simulink model "Modelo_Sensores_Ancho_banda_limitado"  (R2017a)
settings: Solver=VariableStepAuto  StartTime=0.0  StopTime=25  RelTol=1e-3
values from neighbouring files (symbols this model uses):
  alfa_cu = 3.9e-3    (= 0.0039)    [modelo_global_NL.m]
  ba = Jeq*n*wpos    (= 0.0113117692401)    [modelo_global_NL.m]
  beq = bl/r^2 + bm    (= 1.5638971155e-05)    [Evaluacion_polos_5_2_2.m]    (also in modelo_global_NL.m = 1.5e-05)
  Cts = 0.818    [modelo_global_NL.m]
  den_iabc = [1 2*wn_iabc*xita_iabc wn_iabc^2]    [modelo_global_NL.m]
  den_t = [1 2*wn_t*xita_t wn_t^2]    [modelo_global_NL.m]
  den_temp = [tau 1]    [modelo_global_NL.m]
  Jeq = Jl/r^2 + Jm    (= 6.9338269301e-06)    [Evaluacion_polos_5_2_2.m]    (also in modelo_global_NL.m = 5.65588462007e-06)
  ki = 6.5536e10    (= 65536000000)    [modelo_global_NL.m]
  Ksa = Jeq*n*wpos^2    (= 9.04941539211)    [modelo_global_NL.m]
  Ksia = Jeq*wpos^3    (= 2895.81292547)    [modelo_global_NL.m]
  kt = 12800    [modelo_global_NL.m]
  kw = 5.12e7    (= 51200000)    [modelo_global_NL.m]
  LambdaM = 0.01546    [Evaluacion_polos_5_2_2.m]    (also in modelo_global_NL.m)
  Ld = 0.0066    [Evaluacion_polos_5_2_2.m]    (also in modelo_global_NL.m)
  Lq = 0.0058    [Evaluacion_polos_5_2_2.m]    (also in modelo_global_NL.m)
  num_iabc = [wn_iabc^2]    [modelo_global_NL.m]
  num_t = [wn_t^2]    [modelo_global_NL.m]
  num_temp = [1]    [modelo_global_NL.m]
  Pp = 3    [Evaluacion_polos_5_2_2.m]    (also in modelo_global_NL.m)
  r = 314    [Evaluacion_polos_5_2_2.m]    (also in modelo_global_NL.m)
  R0 = 4    [Evaluacion_polos_5_2_2.m]    (also in modelo_global_NL.m)
  Rd = 33    [Evaluacion_polos_5_2_2.m]    (also in modelo_global_NL.m)
  Rq = 29    [Evaluacion_polos_5_2_2.m]    (also in modelo_global_NL.m)
  Rs = 1.02    [Evaluacion_polos_5_2_2.m]    (also in modelo_global_NL.m)
  Rsref = 1.02    [modelo_global_NL.m]
  Rts_amb = 146.7    [modelo_global_NL.m]
  Tamb = 40    [modelo_global_NL.m]
  Tleq = Tl/r    (= 0.02)    [modelo_global_NL.m]
  Tsref = 40    [modelo_global_NL.m]
undefined symbols (not defined in the file or in its folder): sigbuilder_block
settings Model: Creator=merem  LastModifiedBy=merem

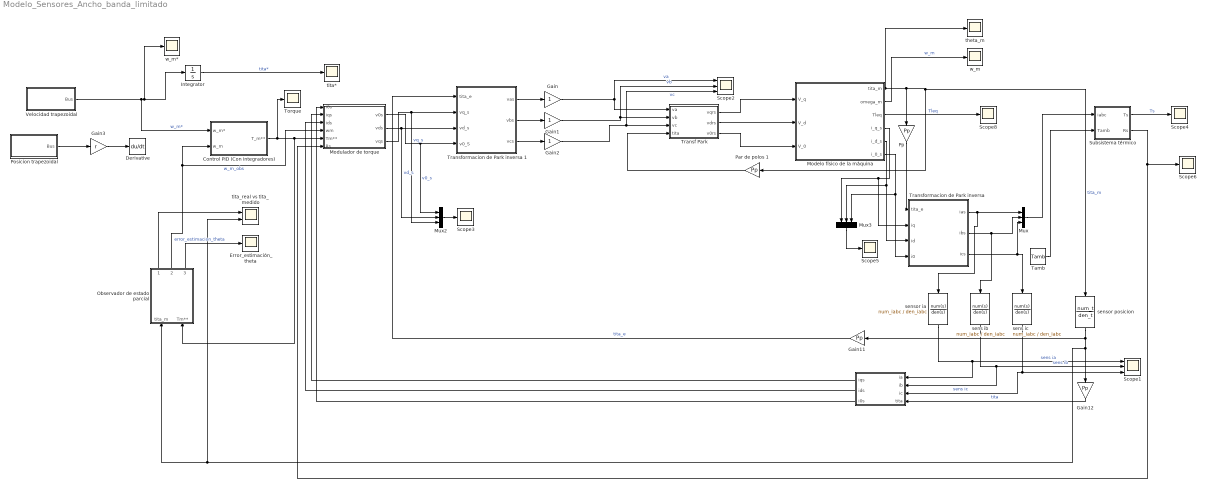
== system Modelo_Sensores_Ancho_banda_limitado ==
  " " : Subsystem
  Control PID (Con integradores) : Subsystem
  Derivative : Derivative
  Error_estimación_theta : Scope
  Gain : Gain
  Gain1 : Gain
  Gain11 : Gain  Gain=Pp
  Gain12 : Gain  Gain=Pp
  Gain2 : Gain
  Gain3 : Gain  Gain=r
  Integrator : Integrator
  Modelo físico de la máquina : Subsystem
  Modulador de torque : Subsystem
  Mux : Mux  Inputs=3
  Mux2 : Mux  Inputs=3
  Mux3 : Mux  Inputs=3
  Observador de estado parcial : Subsystem
  Par de polos 1 : Gain  Gain=Pp
  Posicion trapezoidal : Subsystem  Tag=STV Subsys  LoadFcn=sigbuilder_block('load');  StartFcn=sigbuilder_block('start');  StopFcn=sigbuilder_block('stop');  ClipboardFcn=sigbuilder_block('clipboard');  mask(Sigbuilder block){tuvar=[0:10]}
      mask help: Simulink:masks:SigbuilderBlock_MD
      mask init:
      | if ~strcmp(get_param(bdroot(gcbh),'SimulationStatus'),'stopped') tuvar = sigbuilder_block('maskInit'); end
      settings: CopyFcn=sigbuilder_block('copy');  DeleteFcn=sigbuilder_block('delete');  ModelCloseFcn=sigbuilder_block('modelClose');  PreSaveFcn=sigbuilder_block('preSave');  PauseFcn=sigbuilder_block('pause');  ContinueFcn=sigbuilder_block('continue');  NameChangeFcn=sigbuilder_block('namechange');  OpenFcn=sigbuilder_block('open',[6 30 1012.5 447.75 ]);  CloseFcn=sigbuilder_block('close');
      mask Display: plot(0, 0, 100, 100,[2, 2, 32, 32, 2], [68, 8, 8, 68, 68],[32, 2], [38, 38], [32, 19, 2],[53, 60, 44], [32, 17, 17, 2],[16, 16, 31, 31]);txt = getActiveGroup(gcbh);text(2, 100, txt,'verticalAlignment', 'top');
  Pp : Gain  Gain=Pp
  Scope1 : Scope  NumInputPorts=3
  Scope2 : Scope  NumInputPorts=3
  Scope{3..6,8} (5 alike) : Scope
  Subsistema térmico : Subsystem
  "Tamb " : Constant  Value=Tamb
  Torque : Scope
  "Transf Park " : Subsystem
  "Transformacion de Park inversa " : Subsystem
  Transformacion de Park inversa 1 : Subsystem
  Velocidad trapezoidal : Subsystem  Tag=STV Subsys  LoadFcn=sigbuilder_block('load');  StartFcn=sigbuilder_block('start');  StopFcn=sigbuilder_block('stop');  ClipboardFcn=sigbuilder_block('clipboard');  mask(Sigbuilder block){tuvar=[0:10]}
      mask help: Simulink:masks:SigbuilderBlock_MD
      mask init:
      | if ~strcmp(get_param(bdroot(gcbh),'SimulationStatus'),'stopped') tuvar = sigbuilder_block('maskInit'); end
      settings: CopyFcn=sigbuilder_block('copy');  DeleteFcn=sigbuilder_block('delete');  ModelCloseFcn=sigbuilder_block('modelClose');  PreSaveFcn=sigbuilder_block('preSave');  PauseFcn=sigbuilder_block('pause');  ContinueFcn=sigbuilder_block('continue');  NameChangeFcn=sigbuilder_block('namechange');  OpenFcn=sigbuilder_block('open',[6 30 1012.5 447.75 ]);  CloseFcn=sigbuilder_block('close');
      mask Display: plot(0, 0, 100, 100,[2, 2, 32, 32, 2], [68, 8, 8, 68, 68],[32, 2], [38, 38], [32, 19, 2],[53, 60, 44], [32, 17, 17, 2],[16, 16, 31, 31]);txt = getActiveGroup(gcbh);text(2, 100, txt,'verticalAlignment', 'top');
  sens ib : TransferFcn  Numerator=num_iabc  Denominator=den_iabc
  sens ic : TransferFcn  Numerator=num_iabc  Denominator=den_iabc
  sensor posicion : TransferFcn  Numerator=num_t  Denominator=den_t
  sensor ia : TransferFcn  Numerator=num_iabc  Denominator=den_iabc
  theta_m : Scope
  tita* : Scope
  tita_real vs tita_medido : Scope  NumInputPorts=2
  w_m : Scope
  w_m* : Scope
  wires:
  Observador de estado parcial/3(error_estim) -> Error_estimación_theta/1  "error_estimacion_theta"
  Transformacion de Park inversa 1/3("vcs ") -> Gain2/1
  Gain2/1 -> Scope2/3, "Transf Park "/3(vc)  "vc"
  sensor posicion/1 -> tita_real vs tita_medido/2, Observador de estado parcial/1(tita_m), Gain12/1, Gain11/1
  Gain3/1 -> Derivative/1
  Integrator/1 -> tita*/1  "tita*"
  Transformacion de Park inversa 1/1(vas) -> Gain/1
  Observador de estado parcial/2(w_m_obs) -> Modulador de torque/4(wm), Control PID (Con integradores)/2(w_m)  "w_m_obs"
  Gain11/1 -> Transformacion de Park inversa 1/1(tita_e)  "tita_e"
  Observador de estado parcial/1("tita_obs ") -> tita_real vs tita_medido/1
  Subsistema térmico/1(Ts) -> Scope4/1  "Ts"
  " "/1(iqs) -> Modulador de torque/2(iqs)
  Modulador de torque/1(v0s) -> Mux2/1, Transformacion de Park inversa 1/4("v0_S ")  "v0_s"
  "Transf Park "/3("v0rs ") -> Modelo físico de la máquina/3(V_0)
  Modulador de torque/3(vqs) -> Mux2/3, Transformacion de Park inversa 1/2(vq_s)  "vq_s"
  Control PID (Con integradores)/1(T_m**) -> Torque/1, Modulador de torque/5(Tm**), Observador de estado parcial/2(Tm**)
  Modelo físico de la máquina/4("i_q_s ") -> Mux3/1, "Transformacion de Park inversa "/2(iq)
  "Transformacion de Park inversa "/2(ibs) -> Mux/2, sens ib/1
  "Transf Park "/1(vqrs) -> Modelo físico de la máquina/1(V_q)
  Velocidad trapezoidal/1(Bus) -> Control PID (Con integradores)/1(w_m*), w_m*/1, Integrator/1  "w_m*"
  Transformacion de Park inversa 1/2(vbs) -> Gain1/1
  " "/3("i0s ") -> Modulador de torque/1(i0s)
  Par de polos 1/1 -> "Transf Park "/4(tita)
  Modulador de torque/2(vds) -> Mux2/2, Transformacion de Park inversa 1/3(vd_s)  "vd_s"
  Gain1/1 -> Scope2/2, "Transf Park "/2(vb)  "vb"
  Mux3/1 -> Scope5/1
  "Transformacion de Park inversa "/3("ics ") -> sens ic/1, Mux/3
  sens ic/1 -> " "/3("ic "), Scope1/3  "sens ic"
  Pp/1 -> "Transformacion de Park inversa "/1(tita_e)
  Mux2/1 -> Scope3/1
  Modelo físico de la máquina/6("i_0_s ") -> Mux3/3, "Transformacion de Park inversa "/4(i0)
  "Transformacion de Park inversa "/1(ias) -> sensor ia/1, Mux/1
  Modelo físico de la máquina/5("i_d_s ") -> Mux3/2, "Transformacion de Park inversa "/3(id)
  sensor ia/1 -> Scope1/1, " "/1("ia ")  "sens ia"
  "Tamb "/1 -> Subsistema térmico/2("Tamb ")
  Modelo físico de la máquina/1("tita_m ") -> theta_m/1, sensor posicion/1, Par de polos 1/1, Pp/1  "tita_m"
  Posicion trapezoidal/1(Bus) -> Gain3/1
  Modelo físico de la máquina/3(Tleq) -> Scope8/1  "Tleq"
  Gain12/1 -> " "/4("tita ")  "tita"
  "Transf Park "/2("vdrs ") -> Modelo físico de la máquina/2(V_d)
  Modelo físico de la máquina/2("omega_m ") -> w_m/1  "w_m"
  Mux/1 -> Subsistema térmico/1(iabc)
  " "/2("ids ") -> Modulador de torque/3(ids)
  Gain/1 -> Scope2/1, "Transf Park "/1("va ")  "va"
  sens ib/1 -> Scope1/2, " "/2("ib ")  "sens ib"
  Subsistema térmico/2(Rs) -> Scope6/1, Modulador de torque/6(Rs)

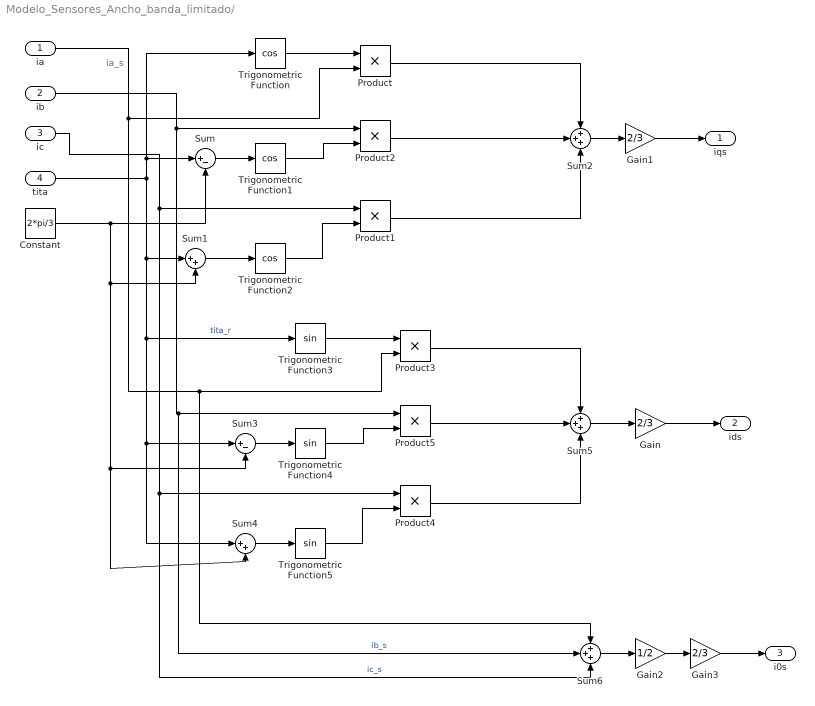
== system Modelo_Sensores_Ancho_banda_limitado/  ==
  note: ia_s
  "ia " : Inport
  "ib " : Inport  Port=2
  "ic " : Inport  Port=3
  "tita " : Inport  Port=4
  Constant : Constant  Value=2*pi/3
  Gain : Gain  Gain=2/3
  Gain1 : Gain  Gain=2/3
  Gain2 : Gain  Gain=1/2
  Gain3 : Gain  Gain=2/3
  Product{,1..5} (6 alike) : Product
  Sum : Sum  Inputs=|+-
  Sum1 : Sum  Inputs=|++
  Sum2 : Sum  Inputs=+++
  Sum3 : Sum  Inputs=|+-
  Sum4 : Sum  Inputs=|++
  Sum5 : Sum  Inputs=+++
  Sum6 : Sum  Inputs=+++
  Trigonometric Function : Trigonometry  Operator=cos
  Trigonometric Function1 : Trigonometry  Operator=cos
  Trigonometric Function2 : Trigonometry  Operator=cos
  Trigonometric Function3 : Trigonometry
  Trigonometric Function4 : Trigonometry
  Trigonometric Function5 : Trigonometry
  iqs : Outport
  "ids " : Outport  Port=2
  "i0s " : Outport  Port=3
  wires:
  "tita "/1 -> Trigonometric Function/1, Sum/1, Sum1/1, Trigonometric Function3/1, Sum3/1, Sum4/1  "tita_r"
  Trigonometric Function/1 -> Product/1
  "ia "/1 -> Sum6/1, Product3/2, Product/2
  Constant/1 -> Sum4/2, Sum3/2, Sum1/2, Sum/2
  Sum/1 -> Trigonometric Function1/1
  Sum1/1 -> Trigonometric Function2/1
  Trigonometric Function1/1 -> Product2/2
  Trigonometric Function2/1 -> Product1/2
  "ib "/1 -> Sum6/2, Product5/1, Product2/1  "ib_s"
  "ic "/1 -> Sum6/3, Product4/1, Product1/1  "ic_s"
  Product/1 -> Sum2/1
  Product2/1 -> Sum2/2
  Sum2/1 -> Gain1/1
  Trigonometric Function5/1 -> Product4/2
  Trigonometric Function3/1 -> Product3/1
  Sum4/1 -> Trigonometric Function5/1
  Sum3/1 -> Trigonometric Function4/1
  Trigonometric Function4/1 -> Product5/2
  Product3/1 -> Sum5/1
  Product5/1 -> Sum5/2
  Product4/1 -> Sum5/3
  Sum5/1 -> Gain/1
  Product1/1 -> Sum2/3
  Gain/1 -> "ids "/1
  Gain1/1 -> iqs/1
  Sum6/1 -> Gain2/1
  Gain2/1 -> Gain3/1
  Gain3/1 -> "i0s "/1

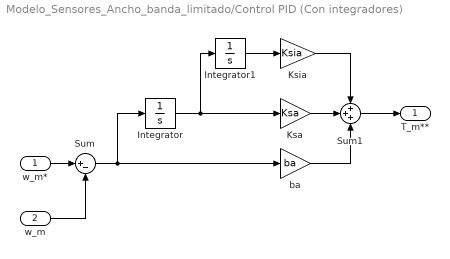
== system Modelo_Sensores_Ancho_banda_limitado/Control PID (Con integradores) ==
  w_m* : Inport
  w_m : Inport  Port=2
  Integrator : Integrator
  Integrator1 : Integrator
  Ksa : Gain  Gain=Ksa
  Ksia : Gain  Gain=Ksia
  Sum : Sum  Inputs=|+-
  Sum1 : Sum  Inputs=+++
  ba : Gain  Gain=ba
  T_m** : Outport
  wires:
  w_m*/1 -> Sum/1
  w_m/1 -> Sum/2
  Sum/1 -> ba/1, Integrator/1
  Integrator/1 -> Integrator1/1, Ksa/1
  Ksa/1 -> Sum1/2
  ba/1 -> Sum1/3
  Ksia/1 -> Sum1/1
  Sum1/1 -> T_m**/1
  Integrator1/1 -> Ksia/1

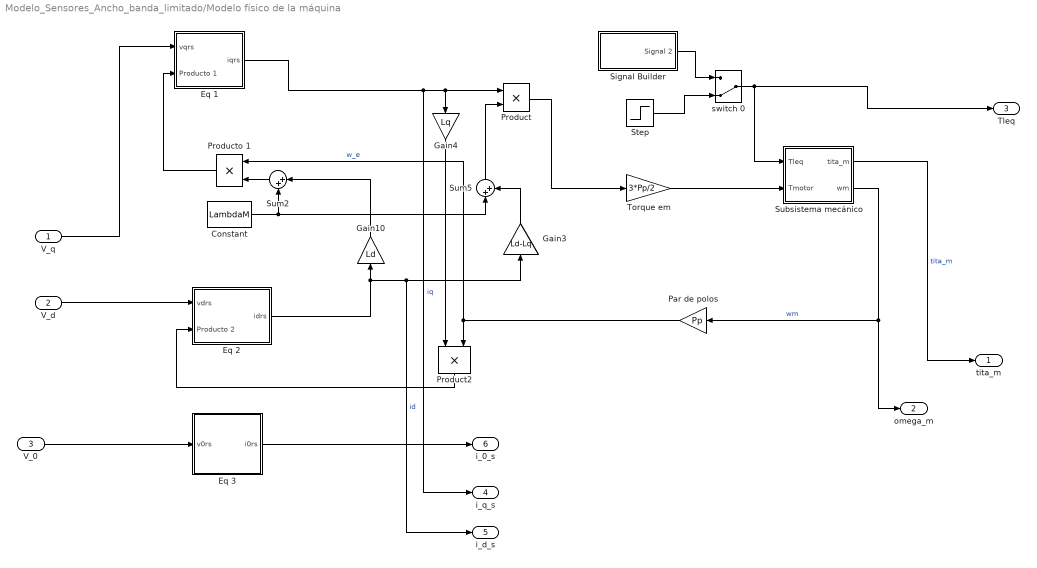
== system Modelo_Sensores_Ancho_banda_limitado/Modelo físico de la máquina ==
  V_q : Inport
  V_d : Inport  Port=2
  V_0 : Inport  Port=3
  Constant : Constant  Value=LambdaM
  Eq 1 : Subsystem
  "Eq 2 " : Subsystem
  Eq 3 : Subsystem
  Gain10 : Gain  Gain=Ld
  Gain3 : Gain  Gain=Ld-Lq
  Gain4 : Gain  Gain=Lq
  Par de polos : Gain  Gain=Pp
  Product : Product
  Product2 : Product
  Producto 1 : Product
  Signal Builder : Subsystem  Tag=STV Subsys  LoadFcn=sigbuilder_block('load');  StartFcn=sigbuilder_block('start');  StopFcn=sigbuilder_block('stop');  ClipboardFcn=sigbuilder_block('clipboard');  mask(Sigbuilder block){tuvar=[0:10]}
      mask help: Simulink:masks:SigbuilderBlock_MD
      mask init:
      | if ~strcmp(get_param(bdroot(gcbh),'SimulationStatus'),'stopped') tuvar = sigbuilder_block('maskInit'); end
      settings: CopyFcn=sigbuilder_block('copy');  DeleteFcn=sigbuilder_block('delete');  ModelCloseFcn=sigbuilder_block('modelClose');  PreSaveFcn=sigbuilder_block('preSave');  PauseFcn=sigbuilder_block('pause');  ContinueFcn=sigbuilder_block('continue');  NameChangeFcn=sigbuilder_block('namechange');  OpenFcn=sigbuilder_block('open',[0 30 1024.5 488.25 ]);  CloseFcn=sigbuilder_block('close');
      mask Display: plot(0, 0, 100, 100,[2, 2, 32, 32, 2], [68, 8, 8, 68, 68],[32, 2], [38, 38], [32, 19, 2],[53, 60, 44], [32, 17, 17, 2],[16, 16, 31, 31]);txt = getActiveGroup(gcbh);text(2, 100, txt,'verticalAlignment', 'top');
  Step : Step  Time=0.3  After=Tleq  SampleTime=0
  Subsistema mecánico : Subsystem
  Sum2 : Sum  Inputs=|++
  Sum5 : Sum  Inputs=|++
  "Torque em " : Gain  Gain=3*Pp/2
  switch 0 : ManualSwitch  CurrentSetting=0
  "tita_m " : Outport
  "omega_m " : Outport  Port=2
  Tleq : Outport  Port=3
  "i_q_s " : Outport  Port=4
  "i_d_s " : Outport  Port=5
  "i_0_s " : Outport  Port=6
  wires:
  Sum2/1 -> Producto 1/2
  Sum5/1 -> Product/2
  Subsistema mecánico/2("wm ") -> "omega_m "/1, Par de polos/1  "wm"
  V_q/1 -> Eq 1/1(vqrs)
  Gain10/1 -> Sum2/1
  Par de polos/1 -> Producto 1/1, Product2/2  "w_e"
  "Torque em "/1 -> Subsistema mecánico/2("Tmotor ")
  Product/1 -> "Torque em "/1
  Constant/1 -> Sum5/1, Sum2/2
  Gain3/1 -> Sum5/2
  Gain4/1 -> Product2/1
  Eq 1/1("iqrs ") -> "i_q_s "/1, Gain4/1, Product/1  "iq"
  Subsistema mecánico/1("tita_m ") -> "tita_m "/1  "tita_m"
  "Eq 2 "/1("idrs ") -> "i_d_s "/1, Gain3/1, Gain10/1  "id"
  Product2/1 -> "Eq 2 "/2("Producto 2 ")
  Producto 1/1 -> Eq 1/2("Producto 1 ")
  V_d/1 -> "Eq 2 "/1("vdrs ")
  V_0/1 -> Eq 3/1("v0rs ")
  Eq 3/1("i0rs ") -> "i_0_s "/1
  Step/1 -> switch 0/2
  switch 0/1 -> Subsistema mecánico/1("Tleq "), Tleq/1
  Signal Builder/1(Signal 2) -> switch 0/1

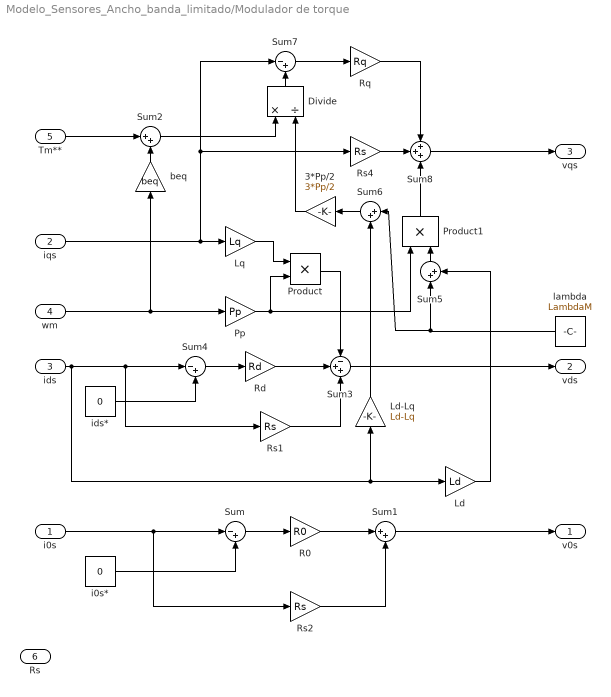
== system Modelo_Sensores_Ancho_banda_limitado/Modulador de torque ==
  i0s : Inport
  iqs : Inport  Port=2
  ids : Inport  Port=3
  wm : Inport  Port=4
  Tm** : Inport  Port=5
  Rs : Inport  Port=6
  3*Pp/2 : Gain  Gain=3*Pp/2
  Divide : Product  Inputs=*/
  Ld : Gain  Gain=Ld
  Ld-Lq : Gain  Gain=Ld-Lq
  Lq : Gain  Gain=Lq
  Pp : Gain  Gain=Pp
  Product : Product
  Product1 : Product
  R0 : Gain  Gain=R0
  Rd : Gain  Gain=Rd
  Rq : Gain  Gain=Rq
  Rs1 : Gain  Gain=Rs
  "Rs2 " : Gain  Gain=Rs
  "Rs4 " : Gain  Gain=Rs
  Sum : Sum  Inputs=|-+
  Sum{1..2,5..6} (4 alike) : Sum  Inputs=|++
  Sum3 : Sum  Inputs=-++
  Sum4 : Sum  Inputs=|-+
  Sum7 : Sum  Inputs=|-+
  Sum8 : Sum  Inputs=+++
  beq : Gain  Gain=beq
  i0s* : Constant  Value=0
  ids* : Constant  Value=0
  lambda : Constant  Value=LambdaM
  v0s : Outport
  vds : Outport  Port=2
  vqs : Outport  Port=3
  wires:
  i0s/1 -> "Rs2 "/1, Sum/1
  Sum1/1 -> v0s/1
  "Rs2 "/1 -> Sum1/2
  R0/1 -> Sum1/1
  Sum/1 -> R0/1
  i0s*/1 -> Sum/2
  Sum3/1 -> vds/1
  Sum4/1 -> Rd/1
  ids/1 -> Ld/1, Ld-Lq/1, Rs1/1, Sum4/1
  ids*/1 -> Sum4/2
  wm/1 -> Pp/1, beq/1
  Pp/1 -> Product1/1, Product/2
  iqs/1 -> "Rs4 "/1, Sum7/1, Lq/1
  Lq/1 -> Product/1
  Rd/1 -> Sum3/2
  Product/1 -> Sum3/1
  Tm**/1 -> Sum2/1
  beq/1 -> Sum2/2
  Sum5/1 -> Product1/2
  Ld/1 -> Sum5/2
  lambda/1 -> Sum5/1, Sum6/1
  Sum6/1 -> 3*Pp/2/1
  Sum2/1 -> Divide/1
  3*Pp/2/1 -> Divide/2
  Sum7/1 -> Rq/1
  Divide/1 -> Sum7/2
  Rq/1 -> Sum8/1
  Product1/1 -> Sum8/3
  Sum8/1 -> vqs/1
  "Rs4 "/1 -> Sum8/2
  Ld-Lq/1 -> Sum6/2
  Rs1/1 -> Sum3/3

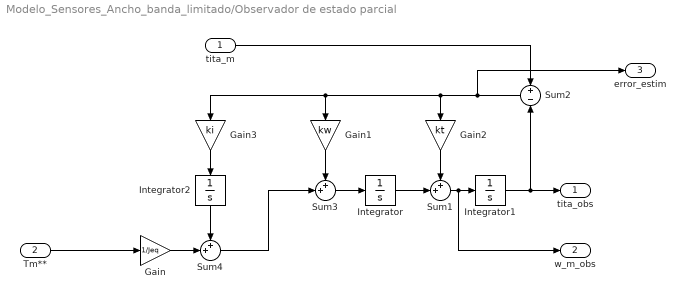
== system Modelo_Sensores_Ancho_banda_limitado/Observador de estado parcial ==
  tita_m : Inport
  Tm** : Inport  Port=2
  Gain : Gain  Gain=1/Jeq
  Gain1 : Gain  Gain=kw
  Gain2 : Gain  Gain=kt
  Gain3 : Gain  Gain=ki
  Integrator : Integrator
  Integrator1 : Integrator
  Integrator2 : Integrator
  Sum1 : Sum  Inputs=++|
  Sum2 : Sum  Inputs=+-
  Sum3 : Sum  Inputs=++|
  Sum4 : Sum  Inputs=++|
  "tita_obs " : Outport
  w_m_obs : Outport  Port=2
  error_estim : Outport  Port=3
  wires:
  Tm**/1 -> Gain/1
  Sum3/1 -> Integrator/1
  Integrator1/1 -> "tita_obs "/1, Sum2/2
  tita_m/1 -> Sum2/1
  Sum2/1 -> error_estim/1, Gain2/1, Gain1/1, Gain3/1
  Gain2/1 -> Sum1/1
  Integrator/1 -> Sum1/2
  Gain1/1 -> Sum3/1
  Sum1/1 -> w_m_obs/1, Integrator1/1
  Gain3/1 -> Integrator2/1
  Sum4/1 -> Sum3/2
  Gain/1 -> Sum4/2
  Integrator2/1 -> Sum4/1

== system Modelo_Sensores_Ancho_banda_limitado/Posicion trapezoidal ==
  Bus Creator : BusCreator  Tag=Bus Creator  Inputs=1
  FromWs : FromWorkspace  Tag=STV FromWs  VariableName=tuvar  SampleTime=0
      SigBuilderData=|
      | common.afterFinalStr = 'Extrapolate'
      | common.sampleTime = 0
      | dataSet.timeRange = [0 25]
      | dataSet.name = 'Group 1'
      | sbobj.Groups.Name = 'Group 1'
      | sbobj.Groups.Signals.Name = 'Signal 2'
      | sbobj.Groups.Signals.XData = [0 4 5 10 15 20 25]
      | sbobj.Groups.Signals.YData = [0 0 0 6.28 6.28 0 0]
      | sbobj.Groups.TimeRange = [0 25]
  Subsystem : Subsystem
  Bus : Outport
  wires:
  FromWs/1 -> Subsystem/1(In1)
  Bus Creator/1 -> Bus/1
  Subsystem/1(Signal 2) -> Bus Creator/1  "Signal 2"

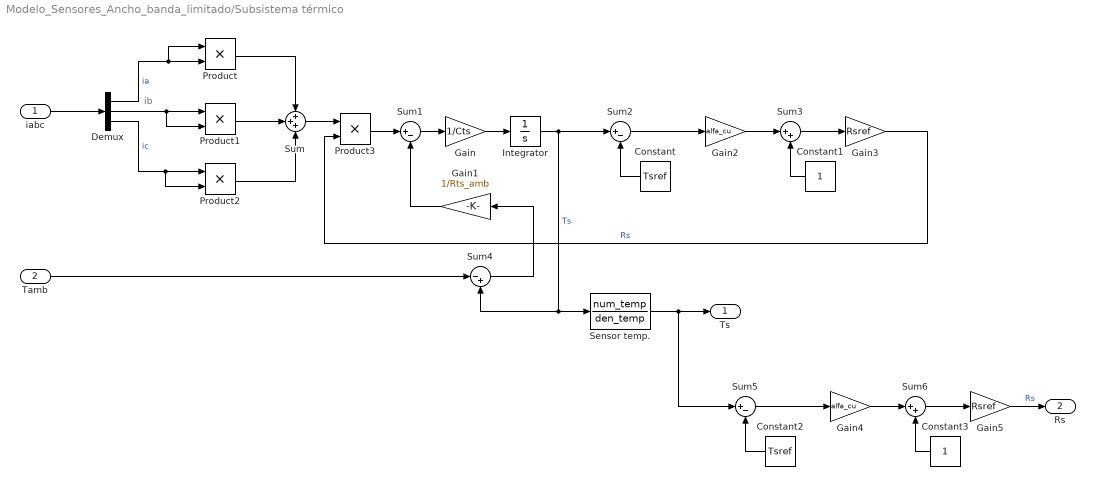
== system Modelo_Sensores_Ancho_banda_limitado/Subsistema térmico ==
  note: ib
  iabc : Inport
  "Tamb " : Inport  Port=2
  Constant : Constant  Value=Tsref
  Constant1 : Constant
  Constant2 : Constant  Value=Tsref
  Constant3 : Constant
  Demux : Demux  Outputs=3
  Gain : Gain  Gain=1/Cts
  Gain1 : Gain  Gain=1/Rts_amb
  Gain2 : Gain  Gain=alfa_cu
  Gain3 : Gain  Gain=Rsref
  Gain4 : Gain  Gain=alfa_cu
  Gain5 : Gain  Gain=Rsref
  Integrator : Integrator  InitialCondition=40
  Product{,1..3} (4 alike) : Product
  Sensor temp. : TransferFcn  Numerator=num_temp  Denominator=den_temp
  Sum : Sum  Inputs=+++
  Sum1 : Sum  Inputs=|+-
  Sum2 : Sum  Inputs=|+-
  Sum3 : Sum  Inputs=|++
  Sum4 : Sum  Inputs=|-+
  Sum5 : Sum  Inputs=|+-
  Sum6 : Sum  Inputs=|++
  Ts : Outport
  Rs : Outport  Port=2
  wires:
  iabc/1 -> Demux/1
  Demux/1 -> Product/2, Product/1  "ia"
  Demux/2 -> Product1/2, Product1/1
  Demux/3 -> Product2/2, Product2/1  "ic"
  Product/1 -> Sum/1
  Product1/1 -> Sum/2
  Product2/1 -> Sum/3
  Sum/1 -> Product3/1
  Gain/1 -> Integrator/1
  Product3/1 -> Sum1/1
  Sum1/1 -> Gain/1
  Gain1/1 -> Sum1/2
  Integrator/1 -> Sensor temp./1, Sum4/2, Sum2/1  "Ts"
  Constant/1 -> Sum2/2
  Sum2/1 -> Gain2/1
  Gain2/1 -> Sum3/1
  Constant1/1 -> Sum3/2
  Sum3/1 -> Gain3/1
  Gain3/1 -> Product3/2  "Rs"
  "Tamb "/1 -> Sum4/1
  Sum4/1 -> Gain1/1
  Sensor temp./1 -> Sum5/1, Ts/1
  Gain4/1 -> Sum6/1
  Sum5/1 -> Gain4/1
  Sum6/1 -> Gain5/1
  Constant2/1 -> Sum5/2
  Constant3/1 -> Sum6/2
  Gain5/1 -> Rs/1  "Rs"

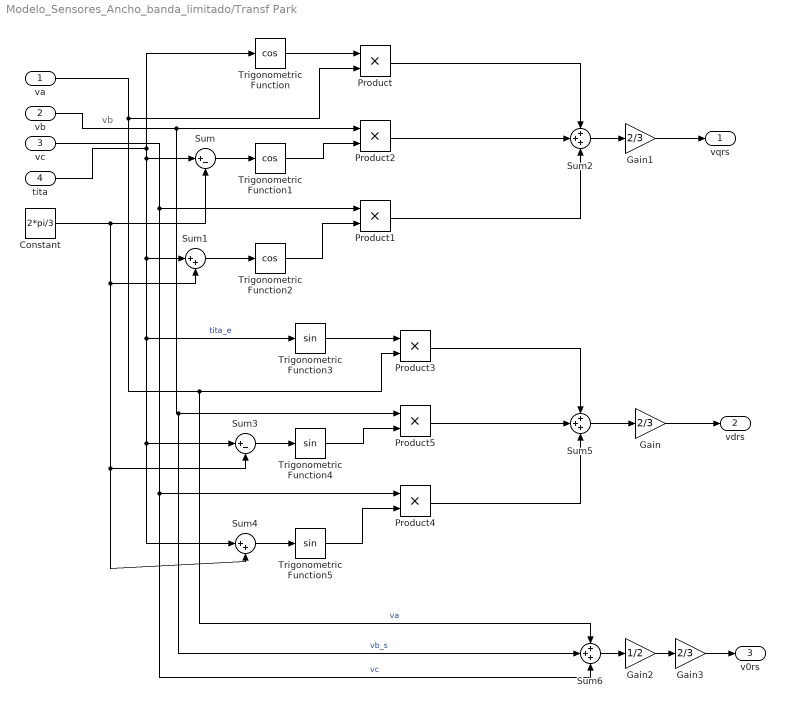
== system Modelo_Sensores_Ancho_banda_limitado/Transf Park  ==
  note: vb
  "va " : Inport
  vb : Inport  Port=2
  vc : Inport  Port=3
  tita : Inport  Port=4
  Constant : Constant  Value=2*pi/3
  Gain : Gain  Gain=2/3
  Gain1 : Gain  Gain=2/3
  Gain2 : Gain  Gain=1/2
  Gain3 : Gain  Gain=2/3
  Product{,1..5} (6 alike) : Product
  Sum : Sum  Inputs=|+-
  Sum1 : Sum  Inputs=|++
  Sum2 : Sum  Inputs=+++
  Sum3 : Sum  Inputs=|+-
  Sum4 : Sum  Inputs=|++
  Sum5 : Sum  Inputs=+++
  Sum6 : Sum  Inputs=+++
  Trigonometric Function : Trigonometry  Operator=cos
  Trigonometric Function1 : Trigonometry  Operator=cos
  Trigonometric Function2 : Trigonometry  Operator=cos
  Trigonometric Function3 : Trigonometry
  Trigonometric Function4 : Trigonometry
  Trigonometric Function5 : Trigonometry
  vqrs : Outport
  "vdrs " : Outport  Port=2
  "v0rs " : Outport  Port=3
  wires:
  tita/1 -> Sum1/1, Trigonometric Function3/1, Sum3/1, Sum4/1, Sum/1, Trigonometric Function/1  "tita_e"
  Trigonometric Function/1 -> Product/1
  "va "/1 -> Sum6/1, Product3/2, Product/2  "va"
  Constant/1 -> Sum4/2, Sum3/2, Sum1/2, Sum/2
  Sum/1 -> Trigonometric Function1/1
  Sum1/1 -> Trigonometric Function2/1
  Trigonometric Function1/1 -> Product2/2
  Trigonometric Function2/1 -> Product1/2
  vb/1 -> Sum6/2, Product5/1, Product2/1  "vb_s"
  vc/1 -> Sum6/3, Product4/1, Product1/1  "vc"
  Product/1 -> Sum2/1
  Product2/1 -> Sum2/2
  Sum2/1 -> Gain1/1
  Trigonometric Function5/1 -> Product4/2
  Trigonometric Function3/1 -> Product3/1
  Sum4/1 -> Trigonometric Function5/1
  Sum3/1 -> Trigonometric Function4/1
  Trigonometric Function4/1 -> Product5/2
  Product3/1 -> Sum5/1
  Product5/1 -> Sum5/2
  Product4/1 -> Sum5/3
  Sum5/1 -> Gain/1
  Product1/1 -> Sum2/3
  Gain/1 -> "vdrs "/1
  Gain1/1 -> vqrs/1
  Sum6/1 -> Gain2/1
  Gain3/1 -> "v0rs "/1
  Gain2/1 -> Gain3/1

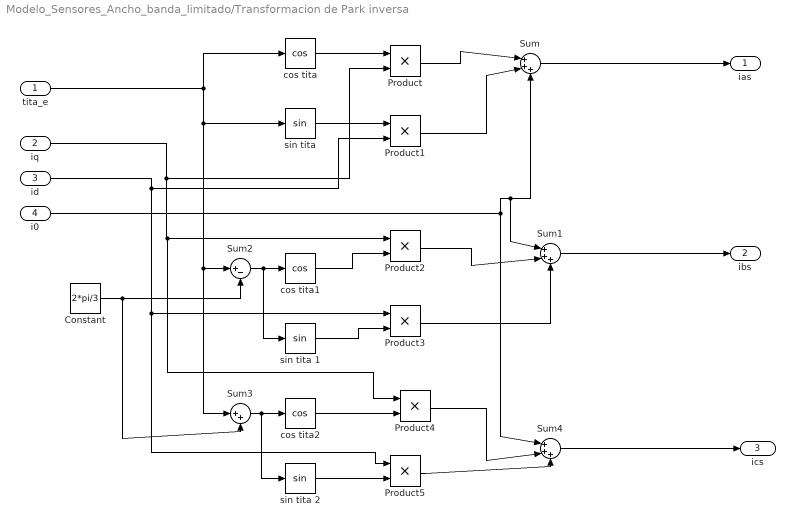
== system Modelo_Sensores_Ancho_banda_limitado/Transformacion de Park inversa  ==
  tita_e : Inport
  iq : Inport  Port=2
  id : Inport  Port=3
  i0 : Inport  Port=4
  Constant : Constant  Value=2*pi/3
  Product{,1..5} (6 alike) : Product
  Sum : Sum  Inputs=|+++
  Sum1 : Sum  Inputs=|+++
  Sum2 : Sum  Inputs=|+-
  Sum3 : Sum  Inputs=|++
  Sum4 : Sum  Inputs=|+++
  cos tita : Trigonometry  Operator=cos
  cos tita1 : Trigonometry  Operator=cos
  cos tita2 : Trigonometry  Operator=cos
  "sin tita " : Trigonometry
  sin tita 1 : Trigonometry
  sin tita 2 : Trigonometry
  ias : Outport
  ibs : Outport  Port=2
  "ics " : Outport  Port=3
  wires:
  tita_e/1 -> Sum3/1, Sum2/1, "sin tita "/1, cos tita/1
  iq/1 -> Product4/1, Product2/1, Product/2
  cos tita/1 -> Product/1
  "sin tita "/1 -> Product1/1
  id/1 -> Product5/1, Product3/1, Product1/2
  Product/1 -> Sum/1
  Product1/1 -> Sum/2
  Sum/1 -> ias/1
  i0/1 -> Sum1/1, Sum/3, Sum4/1
  cos tita1/1 -> Product2/2
  sin tita 1/1 -> Product3/2
  Product3/1 -> Sum1/3
  Product2/1 -> Sum1/2
  Sum1/1 -> ibs/1
  Constant/1 -> Sum3/2, Sum2/2
  Sum2/1 -> sin tita 1/1, cos tita1/1
  Sum3/1 -> sin tita 2/1, cos tita2/1
  cos tita2/1 -> Product4/2
  sin tita 2/1 -> Product5/2
  Product5/1 -> Sum4/3
  Product4/1 -> Sum4/2
  Sum4/1 -> "ics "/1

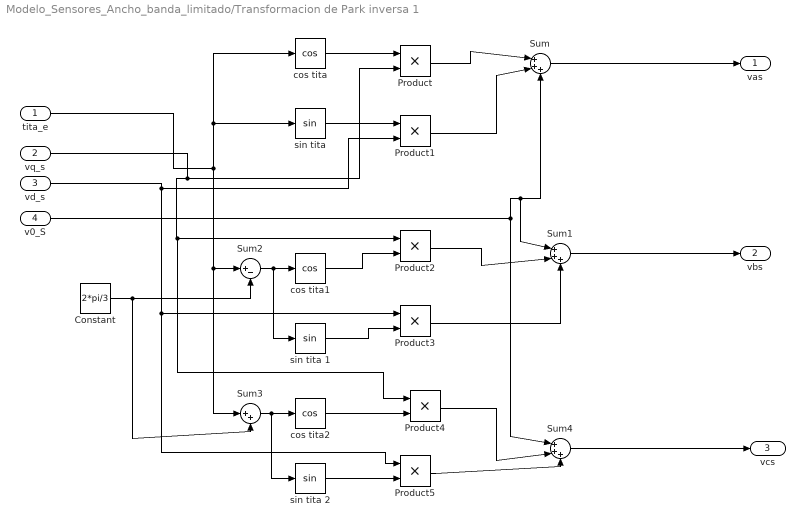
== system Modelo_Sensores_Ancho_banda_limitado/Transformacion de Park inversa 1 ==
  tita_e : Inport
  vq_s : Inport  Port=2
  vd_s : Inport  Port=3
  "v0_S " : Inport  Port=4
  Constant : Constant  Value=2*pi/3
  Product{,1..5} (6 alike) : Product
  Sum : Sum  Inputs=|+++
  Sum1 : Sum  Inputs=|+++
  Sum2 : Sum  Inputs=|+-
  Sum3 : Sum  Inputs=|++
  Sum4 : Sum  Inputs=|+++
  cos tita : Trigonometry  Operator=cos
  cos tita1 : Trigonometry  Operator=cos
  cos tita2 : Trigonometry  Operator=cos
  "sin tita " : Trigonometry
  sin tita 1 : Trigonometry
  sin tita 2 : Trigonometry
  vas : Outport
  vbs : Outport  Port=2
  "vcs " : Outport  Port=3
  wires:
  tita_e/1 -> Sum3/1, Sum2/1, cos tita/1, "sin tita "/1
  vq_s/1 -> Product4/1, Product2/1, Product/2
  cos tita/1 -> Product/1
  "sin tita "/1 -> Product1/1
  vd_s/1 -> Product5/1, Product3/1, Product1/2
  Product/1 -> Sum/1
  Product1/1 -> Sum/2
  Sum/1 -> vas/1
  "v0_S "/1 -> Sum1/1, Sum/3, Sum4/1
  cos tita1/1 -> Product2/2
  sin tita 1/1 -> Product3/2
  Product3/1 -> Sum1/3
  Product2/1 -> Sum1/2
  Sum1/1 -> vbs/1
  Constant/1 -> Sum3/2, Sum2/2
  Sum2/1 -> sin tita 1/1, cos tita1/1
  Sum3/1 -> sin tita 2/1, cos tita2/1
  cos tita2/1 -> Product4/2
  sin tita 2/1 -> Product5/2
  Product5/1 -> Sum4/3
  Product4/1 -> Sum4/2
  Sum4/1 -> "vcs "/1

== system Modelo_Sensores_Ancho_banda_limitado/Velocidad trapezoidal ==
  Bus Creator : BusCreator  Tag=Bus Creator  Inputs=1
  FromWs : FromWorkspace  Tag=STV FromWs  VariableName=tuvar  SampleTime=0
      SigBuilderData=|
      | common.afterFinalStr = 'Extrapolate'
      | common.sampleTime = 0
      | dataSet.timeRange = [0 25]
      | dataSet.name = 'Group 1'
      | sbobj.Groups.Name = 'Group 1'
      | sbobj.Groups.Signals.Name = 'Signal 1'
      | sbobj.Groups.Signals.XData = [0 5 5.497 9.502 10 15 15.49 19.497 20 25]
      | sbobj.Groups.Signals.YData = [0 0 380 380 0 0 -380 -380 0 0]
      | sbobj.Groups.TimeRange = [0 25]
  Subsystem : Subsystem
  Bus : Outport
  wires:
  FromWs/1 -> Subsystem/1(In1)
  Bus Creator/1 -> Bus/1
  Subsystem/1(Signal 1) -> Bus Creator/1  "Signal 1"

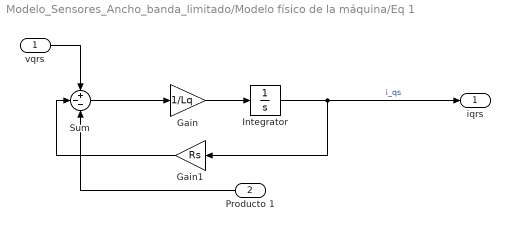
== system Modelo_Sensores_Ancho_banda_limitado/Modelo físico de la máquina/Eq 1 ==
  vqrs : Inport
  "Producto 1 " : Inport  Port=2
  Gain : Gain  Gain=1/Lq
  Gain1 : Gain  Gain=Rs
  Integrator : Integrator
  Sum : Sum  Inputs=+--
  "iqrs " : Outport
  wires:
  Gain/1 -> Integrator/1
  Sum/1 -> Gain/1
  vqrs/1 -> Sum/1
  Gain1/1 -> Sum/2
  "Producto 1 "/1 -> Sum/3
  Integrator/1 -> "iqrs "/1, Gain1/1  "i_qs"

== system Modelo_Sensores_Ancho_banda_limitado/Modelo físico de la máquina/Eq 2  ==
  "vdrs " : Inport
  "Producto 2 " : Inport  Port=2
  Gain11 : Gain  Gain=Rs
  Gain2 : Gain  Gain=1/Ld
  Integrator1 : Integrator
  Sum1 : Sum  Inputs=|+-+
  "idrs " : Outport
  wires:
  "Producto 2 "/1 -> Sum1/3
  Gain2/1 -> Integrator1/1
  Gain11/1 -> Sum1/2
  Sum1/1 -> Gain2/1
  Integrator1/1 -> Gain11/1, "idrs "/1  "i_ds"
  "vdrs "/1 -> Sum1/1

== system Modelo_Sensores_Ancho_banda_limitado/Modelo físico de la máquina/Eq 3 ==
  "v0rs " : Inport
  Gain12 : Gain
  Gain13 : Gain  Gain=Rs
  Integrator5 : Integrator
  Sum4 : Sum  Inputs=|++
  "i0rs " : Outport
  wires:
  Gain12/1 -> Integrator5/1
  Sum4/1 -> Gain12/1
  Gain13/1 -> Sum4/2
  "v0rs "/1 -> Sum4/1
  Integrator5/1 -> "i0rs "/1, Gain13/1  "i_0s"

== system Modelo_Sensores_Ancho_banda_limitado/Modelo físico de la máquina/Signal Builder ==
  Demux : Demux  Tag=STV Demux  Outputs=1
  FromWs : FromWorkspace  Tag=STV FromWs  VariableName=tuvar  SampleTime=0
      SigBuilderData=|
      | common.afterFinalStr = 'Extrapolate'
      | common.sampleTime = 0
      | dataSet.timeRange = [0 2]
      | dataSet.name = 'Group 1'
      | sbobj.Groups.Name = 'Group 1'
      | sbobj.Groups.Signals.Name = 'Signal 2'
      | sbobj.Groups.Signals.XData = [0 0.3 0.3 0.5 0.5 0.9 0.9 2]
      | sbobj.Groups.Signals.YData = [0 0 0.02 0.02 -0.02 -0.02 0 0]
      | sbobj.Groups.TimeRange = [0 2]
  Signal 2 : Outport  Tag=STV Outport
  wires:
  FromWs/1 -> Demux/1
  Demux/1 -> Signal 2/1

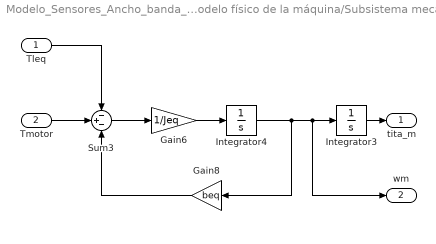
== system Modelo_Sensores_Ancho_banda_limitado/Modelo físico de la máquina/Subsistema mecánico ==
  "Tleq " : Inport
  "Tmotor " : Inport  Port=2
  Gain6 : Gain  Gain=1/Jeq
  Gain8 : Gain  Gain=beq
  Integrator3 : Integrator
  Integrator4 : Integrator
  Sum3 : Sum  Inputs=-+-
  "tita_m " : Outport
  "wm " : Outport  Port=2
  wires:
  Integrator3/1 -> "tita_m "/1
  Integrator4/1 -> Gain8/1, "wm "/1, Integrator3/1
  Sum3/1 -> Gain6/1
  Gain6/1 -> Integrator4/1
  Gain8/1 -> Sum3/3
  "Tleq "/1 -> Sum3/1
  "Tmotor "/1 -> Sum3/2

== system Modelo_Sensores_Ancho_banda_limitado/Posicion trapezoidal/Subsystem ==
  In1 : Inport
  Demux : Demux  Tag=STV Demux  Outputs=1
  Signal 2 : Outport  Tag=STV Outport
  wires:
  In1/1 -> Demux/1
  Demux/1 -> Signal 2/1

== system Modelo_Sensores_Ancho_banda_limitado/Velocidad trapezoidal/Subsystem ==
  In1 : Inport
  Demux : Demux  Tag=STV Demux  Outputs=1
  Signal 1 : Outport  Tag=STV Outport
  wires:
  In1/1 -> Demux/1
  Demux/1 -> Signal 1/1
